simulink model "innerLoop_landing"  (R2024b)
settings: Solver=FixedStepDiscrete  StartTime=0.0  StopTime=0  FixedStep=0.01  RelTol=1e-3
PreLoadFcn:
  | addpath(fileparts(get_param(bdroot,'FileName')));
model workspace (MAT data in the model file):
  H_ship_body = [nan; nan; nan]
  T_body_camera = [nan  nan  nan  nan; nan  nan  nan  nan; nan  nan  nan  nan; nan  nan  nan  nan]
  gear_body = [nan; nan; nan]
undefined symbols (not defined in the file or in its folder): euler_0, V_0
libraries: simulink x1
settings Model: Creator=yuanjiayi  LastModifiedBy=yuanjiayi

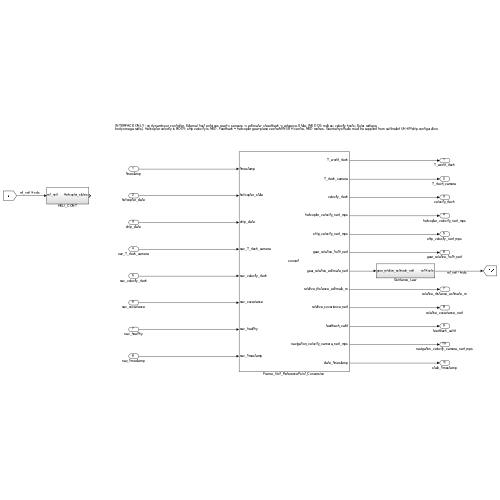
[thumbnail: Simulink's stored preview of the top-level diagram]
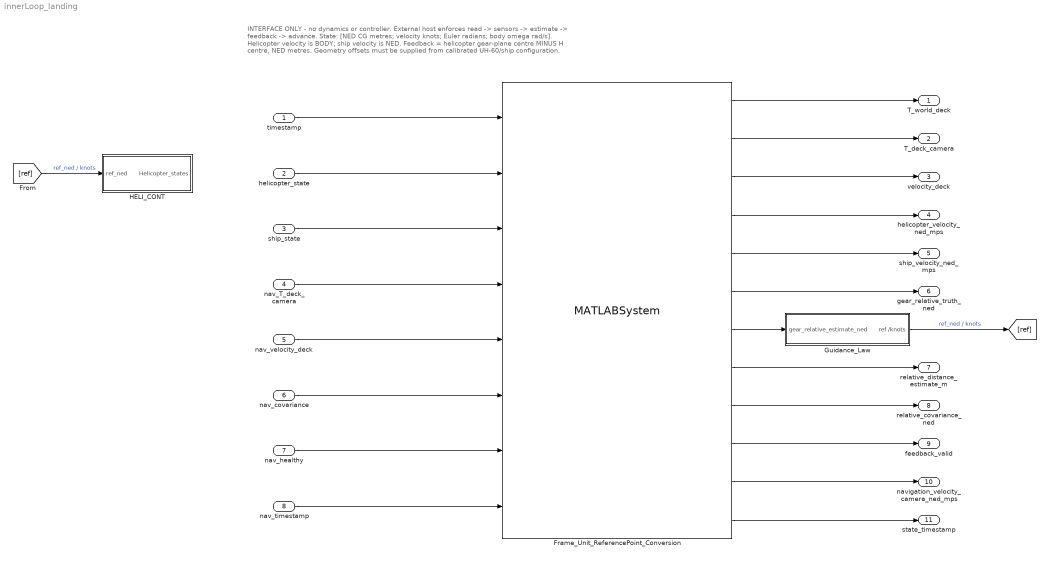
== system innerLoop_landing ==
  note: INTERFACE ONLY - no dynamics or controller. External host enforces read -> sensors -> estimate -> feedback -> advance. State: [NED CG metres; velocity knots; Euler radians;
      | body omega rad/s]. Helicopter velocity is BODY; ship velocity is NED. Feedback = helicopter gear-plane centre MINUS H centre, NED metres. Geometry offsets must be supplied from calibrated UH-60/ship configuration.
  timestamp : Inport  OutDataTypeStr=double  PortDimensions=1
  helicopter_state : Inport  Port=2  OutDataTypeStr=double  PortDimensions=12
  ship_state : Inport  Port=3  OutDataTypeStr=double  PortDimensions=12
  nav_T_deck_camera : Inport  Port=4  OutDataTypeStr=double  PortDimensions=[4 4]
  nav_velocity_deck : Inport  Port=5  OutDataTypeStr=double  PortDimensions=3
  nav_covariance : Inport  Port=6  OutDataTypeStr=double  PortDimensions=[6 6]
  nav_healthy : Inport  Port=7  OutDataTypeStr=double  PortDimensions=1
  nav_timestamp : Inport  Port=8  OutDataTypeStr=double  PortDimensions=1
  Frame_Unit_ReferencePoint_Conversion : MATLABSystem  System=convert  T_body_camera=T_body_camera  H_ship_body=H_ship_body  gear_body=gear_body  SimulateUsing=Interpreted execution
      mask Type: convert
      mask Display:
      | disp('convert');
      | port_label('input',1,'timestamp');
      | port_label('input',2,'helicopter_state');
      | port_label('input',3,'ship_state');
      | port_label('input',4,'nav_T_deck_camera');
      | port_label('input',5,'nav_velocity_deck');
      | port_label('input',6,'nav_covariance');
      | port_label('input',7,'nav_healthy');
      | port_label('input',8,'nav_timestamp');
      | port_label('output',1,'T_world_deck');
      | port_label('output',2,'T_deck_camera');
      | port_label('output',3,'velocity_deck');
      | port_label('output',4,'helicopter_velocity_ned_mps');
      | port_label('output',5,'ship_velocity_ned_mps');
      | port_label('output',6,'gear_relative_truth_ned');
      | port_label('output',7,'gear_relative_estimate_ned');
      | port_label('output',8,'relative_distance_estimate_m');
      | port_label('output',9,'relative_covariance_ned');
      | port_label('output',10,'feedback_valid');
      | port_label('output',11,'navigation_velocity_camera_ned_mps');
      | port_label('output',12,'state_timestamp');
  Guidance_Law : Subsystem
  HELI_CONT : Subsystem
  T_world_deck : Outport
  T_deck_camera : Outport  Port=2
  velocity_deck : Outport  Port=3
  helicopter_velocity_ned_mps : Outport  Port=4
  ship_velocity_ned_mps : Outport  Port=5
  gear_relative_truth_ned : Outport  Port=6
  relative_distance_estimate_m : Outport  Port=7
  relative_covariance_ned : Outport  Port=8
  feedback_valid : Outport  Port=9
  navigation_velocity_camera_ned_mps : Outport  Port=10
  state_timestamp : Outport  Port=11
  wires:
  timestamp/1 -> Frame_Unit_ReferencePoint_Conversion/1
  helicopter_state/1 -> Frame_Unit_ReferencePoint_Conversion/2
  ship_state/1 -> Frame_Unit_ReferencePoint_Conversion/3
  nav_T_deck_camera/1 -> Frame_Unit_ReferencePoint_Conversion/4
  nav_velocity_deck/1 -> Frame_Unit_ReferencePoint_Conversion/5
  nav_covariance/1 -> Frame_Unit_ReferencePoint_Conversion/6
  nav_healthy/1 -> Frame_Unit_ReferencePoint_Conversion/7
  nav_timestamp/1 -> Frame_Unit_ReferencePoint_Conversion/8
  Frame_Unit_ReferencePoint_Conversion/1 -> T_world_deck/1
  Frame_Unit_ReferencePoint_Conversion/2 -> T_deck_camera/1
  Frame_Unit_ReferencePoint_Conversion/3 -> velocity_deck/1
  Frame_Unit_ReferencePoint_Conversion/4 -> helicopter_velocity_ned_mps/1
  Frame_Unit_ReferencePoint_Conversion/5 -> ship_velocity_ned_mps/1
  Frame_Unit_ReferencePoint_Conversion/6 -> gear_relative_truth_ned/1
  Frame_Unit_ReferencePoint_Conversion/8 -> relative_distance_estimate_m/1
  Frame_Unit_ReferencePoint_Conversion/9 -> relative_covariance_ned/1
  Frame_Unit_ReferencePoint_Conversion/10 -> feedback_valid/1
  Frame_Unit_ReferencePoint_Conversion/11 -> navigation_velocity_camera_ned_mps/1
  Frame_Unit_ReferencePoint_Conversion/12 -> state_timestamp/1
  [ref] -> HELI_CONT/1(ref_ned)  "ref_ned / knots"
  Frame_Unit_ReferencePoint_Conversion/7 -> Guidance_Law/1(gear_relative_estimate_ned)
  Guidance_Law/1(ref /knots) -> [ref]  "ref_ned / knots"

== system innerLoop_landing/Guidance_Law ==
  gear_relative_estimate_ned : Inport
  Constant2 : Constant  Value=[30; 0; 0]
  MATLAB System : MATLABSystem  System=uvw_Gen  maxDeltaVel_n=1.5  maxDeltaVel_e=0.5  maxDeltaVel_d=1.5  SimulateUsing=Code generation
      mask Type: uvw_Gen
      mask Display:
      | disp('uvw_Gen');
      | port_label('input',1,'Delta_r');
      | port_label('output',1,'Delta_v');
  Plus1 : Sum
  "SCOPE " : Subsystem
  ref /knots : Outport
  wires:
  Plus1/1 -> ref /knots/1  "ref /knots"
  MATLAB System/1 -> Plus1/1
  Constant2/1 -> Plus1/2
  gear_relative_estimate_ned/1 -> MATLAB System/1, "SCOPE "/1(In1)

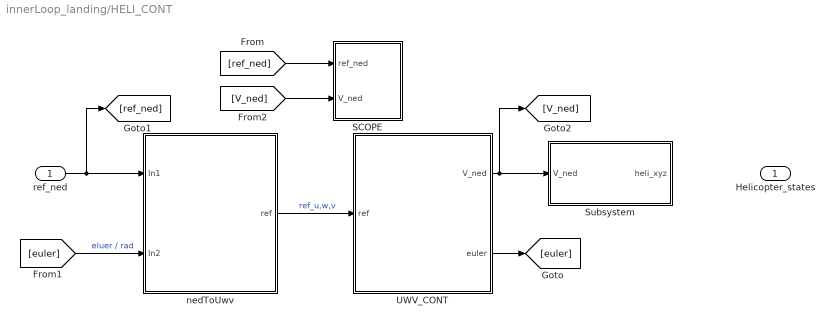
== system innerLoop_landing/HELI_CONT ==
  ref_ned : Inport
  SCOPE : Subsystem
  Subsystem : Subsystem
  UWV_CONT : Subsystem
  nedToUwv : Subsystem
  Helicopter_states : Outport
  wires:
  ref_ned/1 -> [ref_ned], nedToUwv/1(In1)
  UWV_CONT/2(euler) -> [euler]
  UWV_CONT/1(V_ned) -> Subsystem/1(V_ned), [V_ned]
  [euler] -> nedToUwv/2(In2)  "eluer / rad"
  nedToUwv/1(ref) -> UWV_CONT/1(ref)  "ref_u,w,v"
  [ref_ned] -> SCOPE/1(ref_ned)
  [V_ned] -> SCOPE/2(V_ned)

== system innerLoop_landing/Guidance_Law/SCOPE  ==
  In1 : Inport
  Demux : Demux  Outputs=3
  Scope : Scope  NumInputPorts=3
  wires:
  Demux/3 -> Scope/3  "delta_z"
  In1/1 -> Demux/1
  Demux/2 -> Scope/2  "delta_y"
  Demux/1 -> Scope/1  "delta_x"

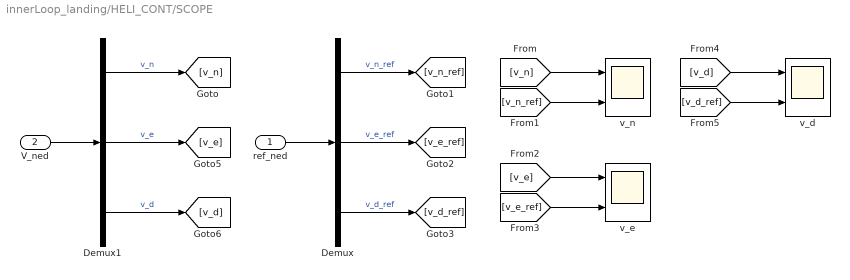
== system innerLoop_landing/HELI_CONT/SCOPE ==
  ref_ned : Inport
  V_ned : Inport  Port=2
  Demux : Demux  Outputs=3
  Demux1 : Demux  Outputs=3
  v_d : Scope  NumInputPorts=2
  v_e : Scope  NumInputPorts=2
  v_n : Scope  NumInputPorts=2
  wires:
  ref_ned/1 -> Demux/1
  V_ned/1 -> Demux1/1
  Demux1/1 -> [v_n]  "v_n"
  Demux/1 -> [v_n_ref]  "v_n_ref"
  [v_n] -> v_n/1
  [v_n_ref] -> v_n/2
  Demux/2 -> [v_e_ref]  "v_e_ref"
  Demux/3 -> [v_d_ref]  "v_d_ref"
  Demux1/2 -> [v_e]  "v_e"
  Demux1/3 -> [v_d]  "v_d"
  [v_e] -> v_e/1
  [v_e_ref] -> v_e/2
  [v_d] -> v_d/1
  [v_d_ref] -> v_d/2

== system innerLoop_landing/HELI_CONT/Subsystem ==
  V_ned : Inport
  Gain : Gain  Gain=0.514444
  Integrator : Integrator  InitialCondition=[0;0;-50]
  heli_xyz : Outport
  wires:
  Integrator/1 -> heli_xyz/1
  V_ned/1 -> Gain/1
  Gain/1 -> Integrator/1

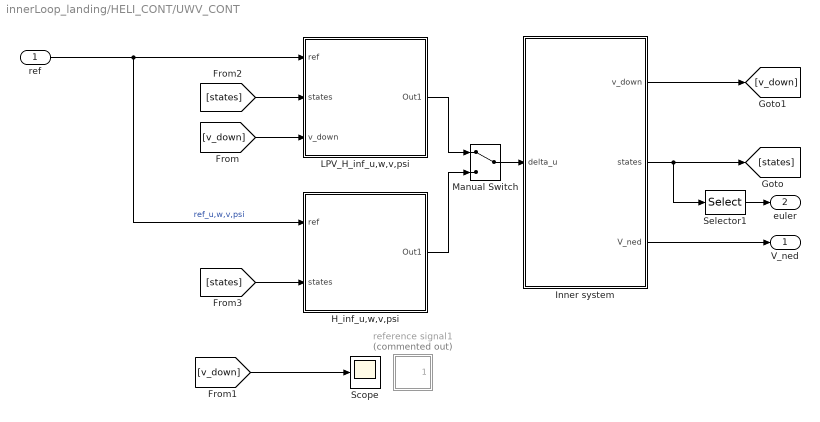
== system innerLoop_landing/HELI_CONT/UWV_CONT ==
  ref : Inport
  H_inf_u,w,v,psi : Subsystem
  Inner system : Subsystem
  LPV_H_inf_u,w,v,psi : Subsystem
  Manual Switch : ManualSwitch
  Scope : Scope
  Selector1 : Selector  InputPortWidth=9  IndexOptions=Index vector (dialog)  Indices=[8 4 9]  OutputSizes=1
  reference signal1 : Subsystem  Commented=on
  V_ned : Outport
  euler : Outport  Port=2
  wires:
  Inner system/1(v_down) -> [v_down]
  Inner system/2(states) -> [states], Selector1/1
  Inner system/3(V_ned) -> V_ned/1
  ref/1 -> H_inf_u,w,v,psi/1(ref), LPV_H_inf_u,w,v,psi/1(ref)  "ref_u,w,v,psi"
  [states] -> LPV_H_inf_u,w,v,psi/2(states)
  [v_down] -> LPV_H_inf_u,w,v,psi/3(v_down)
  [v_down] -> Scope/1
  Selector1/1 -> euler/1
  LPV_H_inf_u,w,v,psi/1(Out1) -> Manual Switch/1
  Manual Switch/1 -> Inner system/1(delta_u)
  H_inf_u,w,v,psi/1(Out1) -> Manual Switch/2
  [states] -> H_inf_u,w,v,psi/2(states)

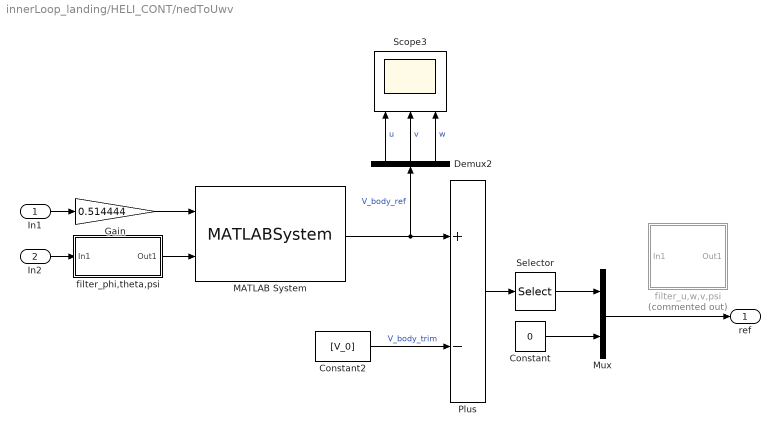
== system innerLoop_landing/HELI_CONT/nedToUwv ==
  In1 : Inport
  In2 : Inport  Port=2
  Constant : Constant  Value=0
  Constant2 : Constant  Value=[V_0]
  Demux2 : Demux  Outputs=3
  Gain : Gain  Gain=0.514444
  MATLAB System : MATLABSystem  System=nedVelToBody  SimulateUsing=Code generation
      mask Type: nedVelToBody
      mask Display:
      | disp('nedVelToBody');
      | port_label('input',1,'V_ned');
      | port_label('input',2,'Euler');
      | port_label('output',1,'V_body');
  Mux : Mux  Inputs=2
  Plus : Sum  Inputs=+-
  Scope3 : Scope  NumInputPorts=3
  Selector : Selector  InputPortWidth=3  IndexOptions=Index vector (dialog)  Indices=[1 3 2]  OutputSizes=1
  filter_phi,theta,psi : Subsystem
  filter_u,w,v,psi : Subsystem  Commented=on
  ref : Outport
  wires:
  filter_phi,theta,psi/1(Out1) -> MATLAB System/2
  Demux2/2 -> Scope3/2  "v"
  Demux2/3 -> Scope3/3  "w"
  In2/1 -> filter_phi,theta,psi/1(In1)
  MATLAB System/1 -> Plus/1, Demux2/1  "V_body_ref"
  Constant/1 -> Mux/2
  In1/1 -> Gain/1
  Demux2/1 -> Scope3/1  "u"
  Plus/1 -> Selector/1
  Constant2/1 -> Plus/2  "V_body_trim"
  Selector/1 -> Mux/1
  Gain/1 -> MATLAB System/1
  Mux/1 -> ref/1

== system innerLoop_landing/HELI_CONT/UWV_CONT/H_inf_u,w,v,psi ==
  ref : Inport
  states : Inport  Port=2
  MATLAB System : MATLABSystem  System=H_inf  PlantA=A_0  PlantB=B_0  ControlledStateIndices=[ 1, 2, 5, 9]  SampleTime=0.02  DKIterations=10  SelectedIteration=6  FrequencyGrid=logspace( -3, 3, 300 )  DiscretizationMethod=tustin  PerformanceA=0.005  PerformanceM=2  PerformanceBandwidth=1  UncertaintyZero=0.2  UncertaintyDenS=0.5  UncertaintyDen0=1  EnableInputSaturation=false  InputLowerLimit=-0.01 * ones( 4, 1 )  InputUpperLimit=0.01 * ones( 4, 1 )  SimulateUsing=Interpreted execution
      mask Type: H_inf
      mask Display:
      | disp('H_inf');
      | port_label('input',1,'r');
      | port_label('input',2,'y');
      | port_label('output',1,'delta');
  SCOPE : Subsystem
  Selector2 : Selector  InputPortWidth=9  IndexOptions=Index vector (dialog)  Indices=[1 2 5 9]  OutputSizes=1
  Out1 : Outport
  wires:
  states/1 -> Selector2/1
  Selector2/1 -> MATLAB System/2, SCOPE/2(y)  "u,w,v,psi"
  MATLAB System/1 -> Out1/1
  ref/1 -> MATLAB System/1, SCOPE/1(ref)

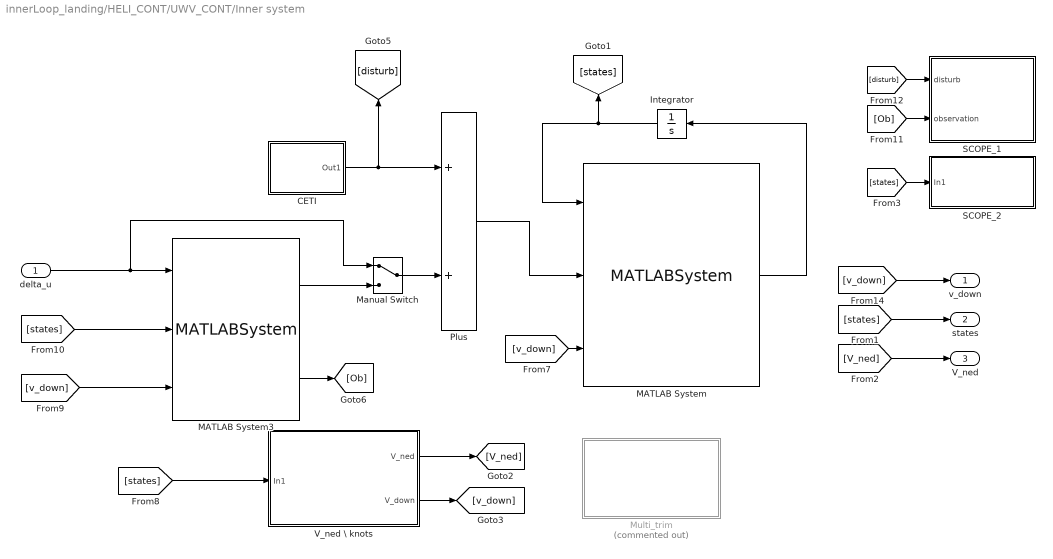
== system innerLoop_landing/HELI_CONT/UWV_CONT/Inner system ==
  delta_u : Inport
  CETI : Subsystem
  Integrator : Integrator  InitialCondition=[0.0;0.0;0.0;0.0;0.0;0.0;0.0;0.0;0.0]
  MATLAB System : MATLABSystem  System=multi_lin_sys  A_10=A_10  B_10=B_10  A_5=A_5  B_5=B_5  A_0=A_0  B_0=B_0  ClampSchedulingVariable=true  SimulateUsing=Interpreted execution
      mask Type: multi_lin_sys
      mask Display:
      | disp('multi_lin_sys');
      | port_label('input',1,'x');
      | port_label('input',2,'delta');
      | port_label('input',3,'v_down');
      | port_label('output',1,'x_dot');
  MATLAB System3 : MATLABSystem  System=LPV_NDO  A_10=A_10  B_10=B_5  A_5=A_5  B_5=B_5  A_0=A_0  B_0=B_0  SampleTime=0.02  ObserverBandwidth=50  ObserverGain_10=[]  ObserverGain_5=[]  ObserverGain_0=[]  DisturbanceFilterBandwidth=0  EnableDisturbanceLimit=true  DisturbanceLowerLimit=[ -0.05; -0.05; -0.05; -0.05 ]  DisturbanceUpperLimit=[ 0.05; 0.05; 0.05; 0.05 ]  EnableInputSaturation=false  InputLowerLimit=[ -inf; -inf; -inf; -inf ]  InputUpperLimit=[ inf; inf; inf; inf ]  ClampSchedulingVariable=true  SimulateUsing=Code generation
      mask Type: LPV_NDO
      mask Display:
      | disp('LPV_NDO');
      | port_label('input',1,'u0');
      | port_label('input',2,'x');
      | port_label('input',3,'v_down');
      | port_label('output',1,'u_comp');
      | port_label('output',2,'d_hat');
  Manual Switch : ManualSwitch
  Multi_trim : Subsystem  Commented=on
  Plus : Sum
  SCOPE_1 : Subsystem
  SCOPE_2 : Subsystem
  V_ned \ knots : Subsystem
  v_down : Outport
  states : Outport  Port=2
  V_ned : Outport  Port=3
  wires:
  [states] -> V_ned \ knots/1(In1)
  [v_down] -> MATLAB System/3
  [states] -> MATLAB System3/2
  MATLAB System/1 -> Integrator/1
  Integrator/1 -> MATLAB System/1, [states]
  CETI/1(Out1) -> Plus/1, [disturb]
  MATLAB System3/2 -> [Ob]
  [v_down] -> MATLAB System3/3
  delta_u/1 -> Manual Switch/1, MATLAB System3/1
  [v_down] -> v_down/1
  [Ob] -> SCOPE_1/2(observation)
  [disturb] -> SCOPE_1/1(disturb)
  [states] -> states/1
  V_ned \ knots/1("V_ned ") -> [V_ned]
  V_ned \ knots/2(V_down) -> [v_down]
  [V_ned] -> V_ned/1
  [states] -> SCOPE_2/1(In1)
  Plus/1 -> MATLAB System/2
  Manual Switch/1 -> Plus/2
  MATLAB System3/1 -> Manual Switch/2

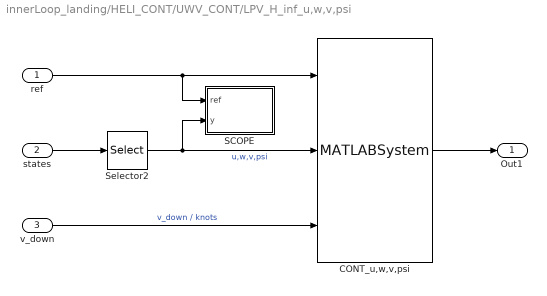
== system innerLoop_landing/HELI_CONT/UWV_CONT/LPV_H_inf_u,w,v,psi ==
  ref : Inport
  states : Inport  Port=2
  v_down : Inport  Port=3
  CONT_u,w,v,psi : MATLABSystem  System=LPV_H_inf  A_10=A_10  B_10=B_10  A_5=A_5  B_5=B_5  A_0=A_0  B_0=B_0  ControlledStateIndices=[ 1, 2, 5, 9]  SampleTime=0.02  DKIterations=10  SelectedIteration=6  FrequencyGrid=logspace( -3, 3, 300 )  DiscretizationMethod=tustin  PerformanceA=0.005  PerformanceM=2  PerformanceBandwidth=1  UncertaintyZero=0.2  UncertaintyDenS=0.5  UncertaintyDen0=1  ClampSchedulingVariable=true  EnableInputSaturation=false  InputLowerLimit=-0.01 * ones( 4, 1 )  InputUpperLimit=0.01 * ones( 4, 1 )  SimulateUsing=Interpreted execution
      mask Type: LPV_H_inf
      mask Display:
      | disp('LPV_H_inf');
      | port_label('input',1,'r');
      | port_label('input',2,'y');
      | port_label('input',3,'v_down');
      | port_label('output',1,'delta');
  SCOPE : Subsystem
  Selector2 : Selector  InputPortWidth=9  IndexOptions=Index vector (dialog)  Indices=[1 2 5 9]  OutputSizes=1
  Out1 : Outport
  wires:
  states/1 -> Selector2/1
  Selector2/1 -> SCOPE/2(y), CONT_u,w,v,psi/2  "u,w,v,psi"
  v_down/1 -> CONT_u,w,v,psi/3  "v_down / knots"
  CONT_u,w,v,psi/1 -> Out1/1
  ref/1 -> SCOPE/1(ref), CONT_u,w,v,psi/1

== system innerLoop_landing/HELI_CONT/UWV_CONT/reference signal1 ==
  Mux : Mux
  Sine Wave : Sin  Amplitude=0.1  Frequency=0.2  SampleTime=0
  Sine Wave1 : Sin  Amplitude=0.1  Frequency=0.15  Phase=pi / 4  SampleTime=0
  Sine Wave2 : Sin  Amplitude=0.1  Frequency=0.15  Phase=pi / 4  SampleTime=0
  Sine Wave3 : Sin  Amplitude=0.0  Frequency=0.15  Phase=pi / 4  SampleTime=0
  Out1 : Outport
  wires:
  Sine Wave/1 -> Mux/1
  Mux/1 -> Out1/1
  Sine Wave1/1 -> Mux/2
  Sine Wave2/1 -> Mux/3
  Sine Wave3/1 -> Mux/4

== system innerLoop_landing/HELI_CONT/nedToUwv/filter_phi,theta,psi ==
  In1 : Inport
  Demux : Demux  Outputs=3
  Mux1 : Mux  Inputs=3
  Transfer Fcn : TransferFcn  Denominator=[10 1]
  Transfer Fcn1 : TransferFcn  Denominator=[10 1]
  Transfer Fcn2 : TransferFcn  Denominator=[10 1]
  Out1 : Outport
  wires:
  Mux1/1 -> Out1/1
  Demux/2 -> Transfer Fcn1/1  "theta"
  Demux/3 -> Transfer Fcn2/1  "psi"
  In1/1 -> Demux/1
  Transfer Fcn1/1 -> Mux1/2  "theta"
  Demux/1 -> Transfer Fcn/1  "phi"
  Transfer Fcn2/1 -> Mux1/3  "psi"
  Transfer Fcn/1 -> Mux1/1  "phi"

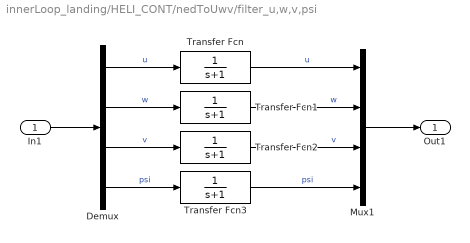
== system innerLoop_landing/HELI_CONT/nedToUwv/filter_u,w,v,psi ==
  In1 : Inport
  Demux : Demux
  Mux1 : Mux
  Transfer Fcn{,1..3} (4 alike) : TransferFcn  Denominator=[1 1]
  Out1 : Outport
  wires:
  Mux1/1 -> Out1/1
  Demux/2 -> Transfer Fcn1/1  "w"
  Transfer Fcn3/1 -> Mux1/4  "psi"
  Demux/4 -> Transfer Fcn3/1  "psi"
  Demux/3 -> Transfer Fcn2/1  "v"
  In1/1 -> Demux/1
  Transfer Fcn1/1 -> Mux1/2  "w"
  Demux/1 -> Transfer Fcn/1  "u"
  Transfer Fcn2/1 -> Mux1/3  "v"
  Transfer Fcn/1 -> Mux1/1  "u"

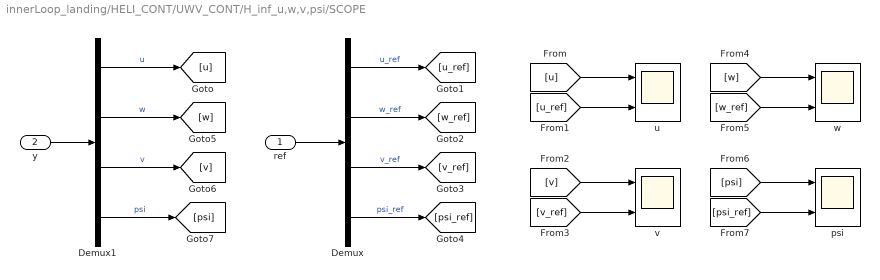
== system innerLoop_landing/HELI_CONT/UWV_CONT/H_inf_u,w,v,psi/SCOPE ==
  ref : Inport
  y : Inport  Port=2
  Demux : Demux
  Demux1 : Demux
  psi : Scope  NumInputPorts=2
  u : Scope  NumInputPorts=2
  v : Scope  NumInputPorts=2
  w : Scope  NumInputPorts=2
  wires:
  ref/1 -> Demux/1
  y/1 -> Demux1/1
  Demux1/1 -> [u]  "u"
  Demux/1 -> [u_ref]  "u_ref"
  [u] -> u/1
  [u_ref] -> u/2
  Demux/2 -> [w_ref]  "w_ref"
  Demux/3 -> [v_ref]  "v_ref"
  Demux/4 -> [psi_ref]  "psi_ref"
  Demux1/2 -> [w]  "w"
  Demux1/3 -> [v]  "v"
  Demux1/4 -> [psi]  "psi"
  [v] -> v/1
  [v_ref] -> v/2
  [w] -> w/1
  [w_ref] -> w/2
  [psi] -> psi/1
  [psi_ref] -> psi/2

== system innerLoop_landing/HELI_CONT/UWV_CONT/Inner system/CETI ==
  Band-Limited White Noise : simulink/Sources/Band-Limited White Noise  Cov=1.0  Ts=0.02  seed=[23341]
  Gain : Gain  Gain=pi / 180
  MATLAB System2 : MATLABSystem  System=CETI  sigma_w=1  Uinf=10  Rm=8.18  Rt=1.68  Ts=0.02  SimulateUsing=Interpreted execution
      mask Type: CETI
      mask Display:
      | disp('CETI');
      | port_label('input',1,'omega_n');
      | port_label('output',1,'du_CETI');
  Out1 : Outport
  wires:
  MATLAB System2/1 -> Gain/1
  Gain/1 -> Out1/1
  Band-Limited White Noise/1 -> MATLAB System2/1

== system innerLoop_landing/HELI_CONT/UWV_CONT/Inner system/Multi_trim ==
  MATLAB System1 : MATLABSystem  System=multi_trim  V_10=V_10  euler_10=euler_10  V_5=V_5  euler_5=euler_5  V_0=V_0  euler_0=euler_0  ClampSchedulingVariable=true  SimulateUsing=Interpreted execution
      mask Type: multi_trim
      mask Display:
      | disp('multi_trim');
      | port_label('input',1,'v_down');
      | port_label('output',1,'trimPos');
  Memory : Memory
  wires:
  MATLAB System1/1 -> [trim]
  [v_down] -> Memory/1
  Memory/1 -> MATLAB System1/1

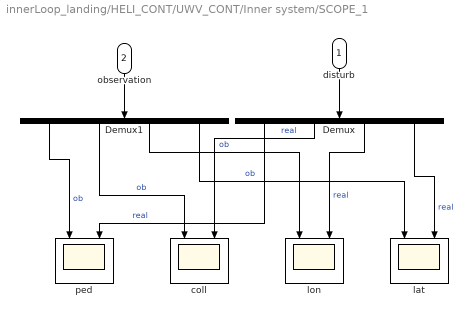
== system innerLoop_landing/HELI_CONT/UWV_CONT/Inner system/SCOPE_1 ==
  disturb : Inport
  observation : Inport  Port=2
  Demux : Demux
  Demux1 : Demux
  coll : Scope  NumInputPorts=2
  lat : Scope  NumInputPorts=2
  lon : Scope  NumInputPorts=2
  ped : Scope  NumInputPorts=2
  wires:
  disturb/1 -> Demux/1
  observation/1 -> Demux1/1
  Demux/4 -> lat/2  "real"
  Demux1/4 -> lat/1  "ob"
  Demux/3 -> lon/2  "real"
  Demux1/3 -> lon/1  "ob"
  Demux/2 -> coll/2  "real"
  Demux1/2 -> coll/1  "ob"
  Demux/1 -> ped/2  "real"
  Demux1/1 -> ped/1  "ob"

== system innerLoop_landing/HELI_CONT/UWV_CONT/Inner system/SCOPE_2 ==
  In1 : Inport
  Demux : Demux  Outputs=9
  delta_states : Scope  NumInputPorts=9
  wires:
  In1/1 -> Demux/1
  Demux/2 -> delta_states/2  "w"
  Demux/6 -> delta_states/6  "p"
  Demux/3 -> delta_states/3  "q"
  Demux/1 -> delta_states/1  "u"
  Demux/5 -> delta_states/5  "v"
  Demux/7 -> delta_states/7  "r"
  Demux/8 -> delta_states/8  "phi"
  Demux/4 -> delta_states/4  "theta"
  Demux/9 -> delta_states/9  "psi"

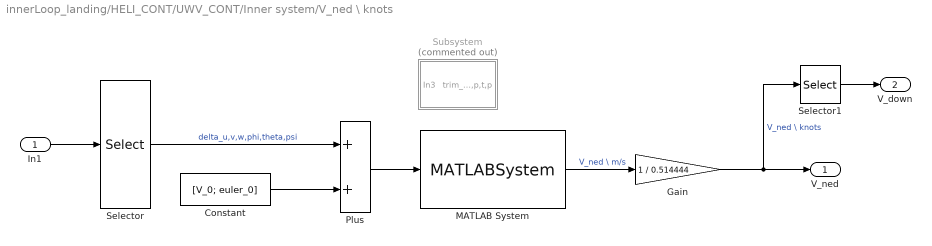
== system innerLoop_landing/HELI_CONT/UWV_CONT/Inner system/V_ned \ knots ==
  In1 : Inport
  Constant : Constant  Value=[V_0; euler_0]
  Gain : Gain  Gain=1 / 0.514444
  MATLAB System : MATLABSystem  System=bodyToNedVel  SimulateUsing=Code generation
      mask Type: bodyToNedVel
      mask Display:
      | disp('bodyToNedVel');
      | port_label('input',1,'states');
      | port_label('output',1,'V_ned');
  Plus : Sum
  Selector : Selector  InputPortWidth=9  IndexOptions=Index vector (dialog)  Indices=[1,5,2,8,4,9]  OutputSizes=1
  Selector1 : Selector  InputPortWidth=3  IndexOptions=Index vector (dialog)  Indices=[3]  OutputSizes=1
  Subsystem : Subsystem  Commented=on
  "V_ned " : Outport
  V_down : Outport  Port=2
  wires:
  In1/1 -> Selector/1
  Constant/1 -> Plus/2
  MATLAB System/1 -> Gain/1  "V_ned \\ m/s"
  Selector/1 -> Plus/1  "delta_u,v,w,phi,theta,psi"
  Gain/1 -> Selector1/1, "V_ned "/1  "V_ned \\ knots"
  Plus/1 -> MATLAB System/1
  Selector1/1 -> V_down/1

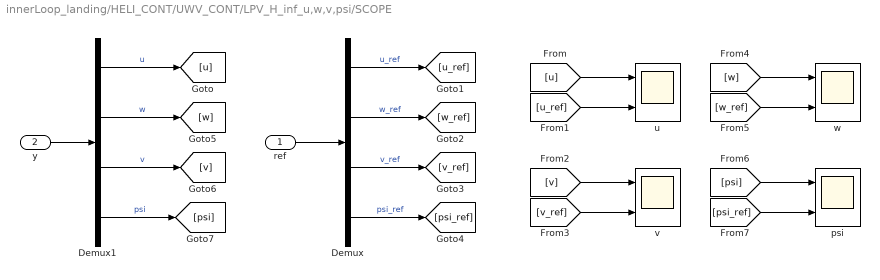
== system innerLoop_landing/HELI_CONT/UWV_CONT/LPV_H_inf_u,w,v,psi/SCOPE ==
  ref : Inport
  y : Inport  Port=2
  Demux : Demux
  Demux1 : Demux
  psi : Scope  NumInputPorts=2
  u : Scope  NumInputPorts=2
  v : Scope  NumInputPorts=2
  w : Scope  NumInputPorts=2
  wires:
  ref/1 -> Demux/1
  y/1 -> Demux1/1
  Demux1/1 -> [u]  "u"
  Demux/1 -> [u_ref]  "u_ref"
  [u] -> u/1
  [u_ref] -> u/2
  Demux/2 -> [w_ref]  "w_ref"
  Demux/3 -> [v_ref]  "v_ref"
  Demux/4 -> [psi_ref]  "psi_ref"
  Demux1/2 -> [w]  "w"
  Demux1/3 -> [v]  "v"
  Demux1/4 -> [psi]  "psi"
  [v] -> v/1
  [v_ref] -> v/2
  [w] -> w/1
  [w_ref] -> w/2
  [psi] -> psi/1
  [psi_ref] -> psi/2

== system innerLoop_landing/HELI_CONT/UWV_CONT/Inner system/V_ned \ knots/Subsystem ==
  In3 : Inport
  MATLAB System1 : MATLABSystem  System=nedVelToBody  SimulateUsing=Code generation
      mask Type: nedVelToBody
      mask Display:
      | disp('nedVelToBody');
      | port_label('input',1,'V_ned');
      | port_label('input',2,'Euler');
      | port_label('output',1,'V_body');
  Mux : Mux  Inputs=2
  "trim : [phi, theta, psi]" : Selector  InputPortWidth=6  IndexOptions=Index vector (dialog)  Indices=[4 5 6]  OutputSizes=1
  "trim : [v_n, v_e, v_d]" : Selector  InputPortWidth=6  IndexOptions=Index vector (dialog)  Indices=[1 2 3]  OutputSizes=1
  trim_u,v,w,p,t,p : Outport
  wires:
  MATLAB System1/1 -> Mux/1  "trim_u,v,w"
  "trim : [phi, theta, psi]"/1 -> MATLAB System1/2, Mux/2  "trim_phi,theta,psi"
  "trim : [v_n, v_e, v_d]"/1 -> MATLAB System1/1
  Mux/1 -> trim_u,v,w,p,t,p/1, [trim]
  In3/1 -> "trim : [phi, theta, psi]"/1, "trim : [v_n, v_e, v_d]"/1
